simulink model "a3e1_2"  (R2020a)
settings: Solver=FixedStepDiscrete  StartTime=0.0  StopTime=10.0  FixedStep=1  RelTol=1e-3
libraries: sldvlib x2, simulink x1
settings Model: Creator=mumun  LastModifiedBy=mumun
settings ConfigComp: DVMode=PropertyProving  DVMaxProcessTime=2000000  DVTestSuiteOptimization=Auto  DVDetectOutOfBounds=on

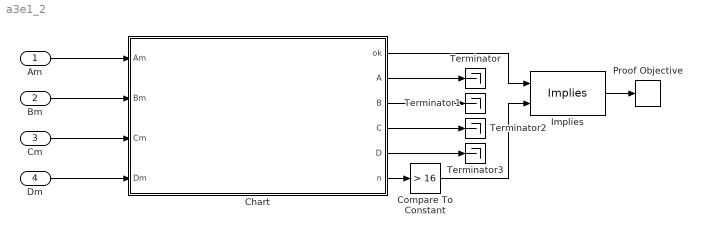
== system a3e1_2 ==
  Am : Inport
  Bm : Inport  Port=2
  Cm : Inport  Port=3
  Dm : Inport  Port=4
  Chart : Stateflow chart  TreatAsAtomicUnit=on
  Compare To Constant : simulink/Logic and Bit Operations/Compare To Constant  relop=>  const=16  OutDataTypeStr=boolean
  Implies : sldvlib/Verification Utilities/Implies
      settings: SourceProductBaseCode=SL
  Proof Objective : sldvlib/Objectives and Constraints/Proof Objective  enabled=on  customAVTBlockType=Proof Objective  intervals=true  dispValues=on  outEnabled=off  enableStopSim=off
      settings: AttributesFormatString=%<intervals>  SourceProductBaseCode=SL
  Terminator{,1..3} (4 alike) : Terminator
  wires:
  Am/1 -> Chart/1(Am)
  Bm/1 -> Chart/2(Bm)
  Cm/1 -> Chart/3(Cm)
  Dm/1 -> Chart/4(Dm)
  Chart/2(A) -> Terminator/1
  Chart/3(B) -> Terminator1/1
  Chart/4(C) -> Terminator2/1
  Chart/5(D) -> Terminator3/1
  Chart/6(n) -> Compare To Constant/1
  Chart/1(ok) -> Implies/1
  Compare To Constant/1 -> Implies/2
  Implies/1 -> Proof Objective/1

== stateflow chart a3e1_2/Chart ==
  settings: executeAtInitialization=1
  state State
  state Goal
  state Complete
  (default) -> State : {A=0;B =0;C =0;D=0;ok=0;n=0;}
  State -> Goal [order 3] : [Dm && !D&&!Cm  && !Bm &&!Am]{D=1; n+=10}
  State -> Goal [order 15] : [Bm && !B&&!Cm && !Dm &&!Am]{B=1; n+=2}
  State -> Goal [order 14] : [Am && !A&& !Cm && !Bm &&!Dm]{A=1; n+=1}
  State -> Goal [order 13] : [Dm && !D && Cm && !C&& !Am && !Bm]{D=1;C=1; n+=10;}
  State -> Goal [order 16] : [Cm && !C&& !Bm && !Am &&!Dm]{C=1; n+=5}
  State -> Goal [order 5] : [Cm && !C&& Bm && !B && !Am && !Dm]{C=1;B=1; n+=5;}
  State -> Goal [order 12] : [Dm && !D && Bm && !B && !Am && !Cm]{D=1;B=1; n+=10;}
  Goal -> State [order 5] : [!Dm && D]{D=0; n+=10;}
  Goal -> State [order 3] : [!Bm && B]{B=0; n+=2;}
  State -> Goal [order 4] : [Bm && !B && Dm && !D && !Cm && !Am]{B=1;D=1; n+=10;}
  Goal -> State [order 2] : [!Am && A]{A=0; n+=1;}
  Goal -> State [order 4] : [!Cm && C]{C=0; n+=5;}
  State -> Goal [order 8] : [Bm && !B && Cm && !C && !Dm && !Am]{B=1;C=1; n+=5;}
  State -> Goal [order 2] : [Am && !A && Bm && !B && !Cm && !Dm]{A=1; B=1; n+=2;}
  State -> Goal [order 6] : [Bm && !B && Am && !A && !Cm && !Dm]{B=1; A=1;n+=2;}
  State -> Goal [order 7] : [Am && !A&& Dm && !D && !Bm && !Cm]{A=1;D=1; n+=10;}
  State -> Goal [order 9] : [Cm && !C && Am && !A && !Dm && !Bm]{C=1;A=1; n+=5;}
  State -> Goal [order 10] : [Cm && !C && Dm && !D && !Am && !Bm]{C=1; D=1;n+=10;}
  State -> Goal [order 11] : [Dm && !D && Am && !A && ! Cm && !Bm]{D=1;A=1; n+=10;}
  State -> Goal [order 1] : [Am && !A&&Cm && !C && !Bm &&!Dm]{A=1;C=1; n+=5}
  Goal -> Complete [order 1] : [A ==1 && B==1 && C==1 && D==1]{ok=1}
  data: ok output boolean; Am input boolean; Bm input boolean; Cm input boolean; Dm input boolean; A output double; B output double; C output double; D output double; n output double
